simulink model "punctdoc"  (Simulink 6.0)
settings: Solver=VariableStepDiscrete  SolverMode=SingleTasking  StartTime=0.0  StopTime=inf  RelTol=1e-3
undefined symbols (not defined in the file or in its folder): figposition, rcosine, slcm
libraries: commsink2 x4, commcnvcod2 x2, dspsigops x2, commsequence2 x2, commdigbbndpm2 x2, dspmlti3 x2, commutil2 x1, commchan2 x1, commrandsrc2 x1
settings Model: RequirementInfo=9  CovMetricSettings=d  Creator=mikem  LastModifiedBy=ysong  ExtModeTrigMode=oneshot  ExtModeArmWhenConnect=off  ExtModeAutoUpdateStatusClock=off
settings DataIOCC: LimitDataPoints=off  SaveOutput=off  SaveTime=off  SignalLoggingName=sigsOut
settings OptimizationCC: BlockReduction=off  BooleanDataType=off  InlineInvariantSignals=off
settings DebuggingCC: CheckExecutionContextPreStartOutputMsg=on  CheckExecutionContextRuntimeOutputMsg=on  SolverPrmCheckMsg=none  InheritedTsInSrcMsg=none  IntegerOverflowMsg=none
settings HardwareCC: TargetUnknown=on
settings ModelReferenceCC: UpdateModelReferenceTargets=IfOutOfDate
settings GRTTargetCC: LifeSpan=inf
settings SFSimCC: SFSimApplyToAllLibs=on  SFSimBuildMode=Incremental

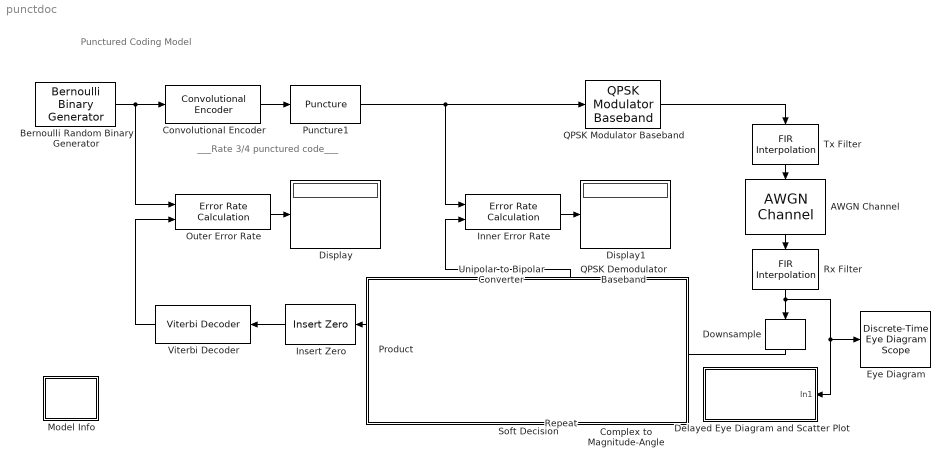
== system punctdoc ==
  note: ___Rate 3/4 punctured code___
  note: Punctured Coding Model
  " Unipolar to Bipolar Converter" : commutil2/Unipolar to Bipolar Converter  Orientation=left  M=2  polarity=Negative
  AWGN Channel : commchan2/AWGN Channel  Orientation=down  seed=123456  noiseMode="Signal to noise ratio  (Es/No)"  EbNodB=10  EsNodB=7  SNRdB=10  bitsPerSym=1  Ps=1/8  Tsym=3/2*5.5e-5  variance=1
  Bernoulli Random Binary Generator : commrandsrc2/Bernoulli Binary Generator  P=0.5  seed=101  Ts=5.5e-5  frameBased=on  sampPerFrame=3  orient=off
  Complex to Magnitude-Angle : ComplexToMagnitudeAngle  Orientation=left  Output=Magnitude
  Convolutional Encoder : commcnvcod2/Convolutional Encoder  trellis=poly2trellis(7, [171 133])  reset=None
  Delayed Eye Diagram and Scatter Plot : Subsystem  Orientation=left  EnableExecutionContextPropagation=on
      mask Display: disp('Delayed Scatter Plot');
  Display : Display
  Display1 : Display
  Downsample : dspsigops/Downsample  Orientation=down  N=8  phase=0  ic=0  smode=Allow multirate  fmode=Maintain input frame size
  "Eye Diagram " : commsink2/Discrete-Time Eye Diagram Scope  Tag=EyeDiagram  sampPerSymb=8  offsetEye=0  symbPerTrace=1  numTraces=40  numNewFrames=10  LineStyles=-  LineColors=r  dupPoints=on  fading=on  render=on  AxisGrid=on  yMin=-1.5  yMax=1.5  inphaseLabel=In-phase Amplitude  quadratureLabel=Quadrature Amplitude  openScopeAtSimStart=off  dispDiagram=In-phase and Quadrature  FrameNumber=off  FigPos=figposition([2.5 55 35 35]);  figTitle=Eye Diagram  block_type_=eye  numLinesMax=50
  Inner Error Rate : commsink2/Error Rate Calculation  N=(3/2+3/2+1)*4  st_delay=0  cp_mode=Entire frame  subframe=[]  PMode=Port  WsName=ErrorVec  RsMode2=off  stop=off  numErr=300  maxBits=1e6
  Insert Zero : commsequence2/Insert Zero  Orientation=left  insertZeroVector=[1 1 0 1 1 0].'
  Model Info : Subsystem  LoadFcn=slcm LoadBlock;  InitFcn=slcm('UpdateAllCMBlocksInThisModelInit')  EnableExecutionContextPropagation=on  mask(CMBlock){InitialSaveTempField=, InitialBlockCM=none, BlockCM=none, Frame=on, SaveTempField=, DisplayStringWithTags=Info, MaskDisplayString=Info, HorizontalTextAlignment=Center, LeftAlignmentValue=0.5, SourceBlockDiagram=punctdoc, TagMaxNumber=20, CMTag1=, CMTag2=, CMTag3=, CMTag4=, CMTag5=, CMTag6=, CMTag7=, CMTag8=, CMTag9=, CMTag10=, CMTag11=, CMTag12=, CMTag13=, CMTag14=, CMTag15=, CMTag16=, CMTag17=, CMTag18=, CMTag19=, CMTag20=}
      mask help: This block allows revision control information to be displayed within the model.
      settings: CopyFcn=slcm CopyBlock;  DeleteFcn=slcm Cancel;  PostSaveFcn=slcm('UpdateAllCMBlocksInThisModel')  NameChangeFcn=slcm Rename;  OpenFcn=commdemohelp;
      mask Display: text(str2num(LeftAlignmentValue), 0.5, MaskDisplayString, 'HorizontalAlignment', HorizontalTextAlignment)
  Outer Error Rate : commsink2/Error Rate Calculation  N=(3/2+3/2+1)*3+96  st_delay=0  cp_mode=Entire frame  subframe=[]  PMode=Port  WsName=ErrorVec  RsMode2=off  stop=on  numErr=50  maxBits=1e6
  Product : Product  Orientation=left  SaturateOnIntegerOverflow=on  InputSameDT=on
  Puncture1 : commsequence2/Puncture  punctureVector=[1 1 0 1 1 0].'
  QPSK Demodulator Baseband : commdigbbndpm2/QPSK Demodulator Baseband  Orientation=left  OutType=Bit  Dec=Gray  Ph=pi/4  numSamp=1
  QPSK Modulator Baseband : commdigbbndpm2/QPSK Modulator Baseband  InType=Bit  Enc=Gray  Ph=pi/4  numSamp=1
  Repeat : dspsigops/Repeat  Orientation=left  N=2  ic=0  mode=Maintain input frame rate
  Rx Filter : dspmlti3/FIR Interpolation  Orientation=down  h=rcosine(1, 8, 'sqrt', 0.5,3)  L=1  framing=Maintain input frame size  outputBufInitCond=0  roundingMode=Floor  overflowMode=off
  Soft Decision : Subsystem  EnableExecutionContextPropagation=on
      mask Display: disp('')
  Tx Filter : dspmlti3/FIR Interpolation  Orientation=down  h=rcosine(1, 8, 'sqrt', 0.5,3)  L=8  framing=Maintain input frame size  outputBufInitCond=0  roundingMode=Floor  overflowMode=off
  Viterbi Decoder : commcnvcod2/Viterbi Decoder  Orientation=left  trellis=poly2trellis(7, [171 133])  dectype=Unquantized  nsdecb=4  tbdepth=96  opmode=Continuous  reset=off
  wires:
  Convolutional Encoder/1 -> Puncture1/1
  Puncture1/1 -> QPSK Modulator Baseband/1, Inner Error Rate/1
  Insert Zero/1 -> Viterbi Decoder/1
  AWGN Channel/1 -> Rx Filter/1
  QPSK Modulator Baseband/1 -> Tx Filter/1
  Complex to Magnitude-Angle/1 -> Repeat/1
  Outer Error Rate/1 -> Display/1
  Inner Error Rate/1 -> Display1/1
  QPSK Demodulator Baseband/1 -> Inner Error Rate/2, " Unipolar to Bipolar Converter"/1
  Product/1 -> Insert Zero/1
  " Unipolar to Bipolar Converter"/1 -> Product/1
  Repeat/1 -> Product/2
  Bernoulli Random Binary Generator/1 -> Convolutional Encoder/1, Outer Error Rate/1
  Viterbi Decoder/1 -> Outer Error Rate/2
  Downsample/1 -> QPSK Demodulator Baseband/1, Complex to Magnitude-Angle/1
  Tx Filter/1 -> AWGN Channel/1
  Rx Filter/1 -> Downsample/1, Delayed Eye Diagram and Scatter Plot/1(In1), "Eye Diagram "/1

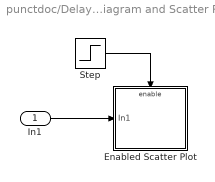
== system punctdoc/Delayed Eye Diagram and Scatter Plot ==
  In1 : Inport  LatchInput=off
  Enabled Scatter Plot : Subsystem  TreatAsAtomicUnit=on  EnableExecutionContextPropagation=on
  Step : Step  Time=3/2*5.5e-5*6  SampleTime=5.5e-5
  wires:
  Step/1 -> Enabled Scatter Plot/Enable
  In1/1 -> Enabled Scatter Plot/1(In1)

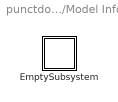
== system punctdoc/Model Info ==
  EmptySubsystem : Subsystem  EnableExecutionContextPropagation=on

== system punctdoc/Soft Decision ==

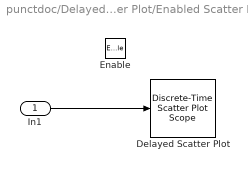
== system punctdoc/Delayed Eye Diagram and Scatter Plot/Enabled Scatter Plot ==
  In1 : Inport  LatchInput=off
  Enable : EnablePort
  "Delayed Scatter Plot " : commsink2/Discrete-Time Scatter Plot Scope  Tag=ScatterPlot  sampPerSymb=8  offsetEye=0  numTraces=1000  numNewFrames=400  LineMarkers=.  LineColors=b  fading=off  render=off  AxisGrid=on  xMin=-1.5  xMax=1.5  yMin=-1.5  yMax=1.5  inphaseLabel=In-phase Amplitude  quadratureLabel=Quadrature Amplitude  openScopeAtSimStart=on  FrameNumber=off  FigPos=[435 333 358 358]  figTitle=Scatter Plot  numLinesMax=50  block_type_=scatter
  wires:
  In1/1 -> "Delayed Scatter Plot "/1

== system punctdoc/Model Info/EmptySubsystem ==
